simulink model "S_ELECTRO2025_V1"  (R2017a)
settings: Solver=VariableStepAuto  StartTime=0.0  StopTime=4  FixedStep=1e-6  MaxStep=1e-4  RelTol=1e-3
values from neighbouring files (symbols this model uses):
  Cdc = 470e-6    (= 0.00047)    [M_ELECTRO2025_V1.m]
  Cpv = 1e-6    (= 1e-06)    [M_ELECTRO2025_V1.m]
  Fred = fs    (= 60)    [M_ELECTRO2025_V1.m]
  fs = 60    [M_ELECTRO2025_V1.m]
  Icc_calc = In/(5/100)    [M_ELECTRO2025_V1.m]
  Irr_in = 0    [M_ELECTRO2025_V1.m]
  K1y2md = Kmd(1:end-1)    [M_ELECTRO2025_V1.m]
  KI2 = Ki2*Ts4    [M_ELECTRO2025_V1.m]
  KI4 = Ki4*Ts4    [M_ELECTRO2025_V1.m]
  KI5 = Ki5*Ts_inv    (= 0.17765287922)    [M_ELECTRO2025_V1.m]
  Kimd = -Kmd(end)    [M_ELECTRO2025_V1.m]
  KP2 = Kp2-KI2/2    [M_ELECTRO2025_V1.m]
  KP4 = Kp4-KI4/2    [M_ELECTRO2025_V1.m]
  KP5 = Kp5*Ts_inv-KI5/2    (= -0.0874937760062)    [M_ELECTRO2025_V1.m]
  L = 68.2729*Lmin    (= 0.100000049318)    [M_ELECTRO2025_V1.m]
  Linv = 0.0133    [M_ELECTRO2025_V1.m]
  Rinv = 0.0417    [M_ELECTRO2025_V1.m]
  S = 10e3*3/2    (= 15000)    [M_ELECTRO2025_V1.m]
  Ts1 = 1/Fs    (= 0.0002)    [M_ELECTRO2025_V1.m]
  Ts4 = 1/(4*Fc)    (= 0.000125)    [M_ELECTRO2025_V1.m]
  Ts_inv = 1/(100*Fc)    (= 5e-06)    [M_ELECTRO2025_V1.m]
  vdc = 1000    [M_ELECTRO2025_V1.m]
  vdc_ref = vdc    (= 1000)    [M_ELECTRO2025_V1.m]
  Vf = VL/sqrt(3)    [M_ELECTRO2025_V1.m]
  VL = (381.051/2)    (= 190.5255)    [M_ELECTRO2025_V1.m]
undefined symbols (not defined in the file or in its folder): DiscIntNeverNeededParam, sigbuilder_block
undefined symbols (not defined in the file): Fs, Ucmax
libraries: powerlib x22, powerlib_meascontrol x10, simulink x3, dsparch4 x3, re_lib x1
settings Model: Creator=dricl  LastModifiedBy=dricl

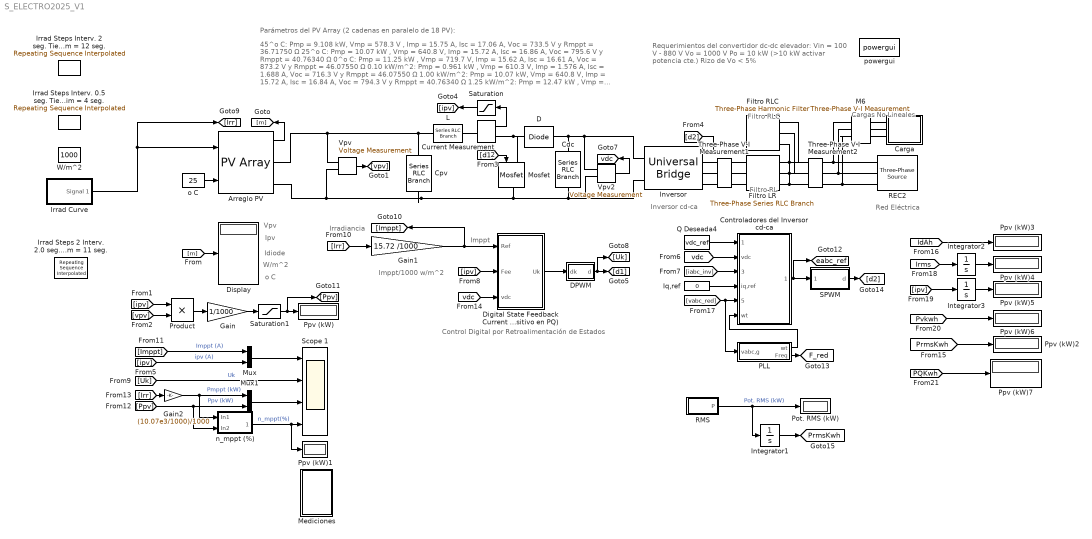
== system S_ELECTRO2025_V1 ==
  note: Control Digital por Retroalimentación de Estados
  note: Irradiancia
  note: Imppt/1000 w/m^2
  note: Imppt
  note: o C
  note: Idiode
  note: Ipv
  note: Vpv
  note: Requerimientos del convertidor dc-dc elevador:
      | Vin = 100 V - 880 V
      | Vo = 1000 V
      | Po = 10 kW (>10 kW activar potencia cte.)
      | Rizo de Vo < 5%
  note: Parámetros del PV Array (2 cadenas en paralelo de 18 PV):
  note: 45^o C: Pmp = 9.108 kW, Vmp = 578.3 V , Imp = 15.75 A, Isc = 17.06 A, Voc = 733.5 V y Rmppt = 36.71750 Ω
      | 25^o C: Pmp = 10.07 kW , Vmp = 640.8 V, Imp = 15.72 A, Isc = 16.86 A, Voc = 795.6 V y Rmppt = 40.76340 Ω
      | 0^o C: Pmp = 11.25 kW , Vmp = 719.7 V, Imp = 15.62 A, Isc = 16.61 A, Voc = 873.2 V y Rmppt = 46.07550 Ω
      | 0.10 kW/m^2: Pmp = 0.961 kW , Vmp = 610.3 V, Imp = 1.576 A, Isc = 1.688 A, Voc = 716.3 V y Rmppt = 46.07550 Ω
      | 1.00 kW/m^2: Pmp = 10.07 kW, Vmp = 640.8 V, Imp = 15.72 A, Isc = 16.84 A, Voc = 794.3 V y Rmppt = 40.76340 Ω
      | 1.25 kW/m^2: Pmp = 12.47 kW , Vmp = 636.0 V, Imp = 19.60 A, Isc = 19.60 A, Voc = 802.6 V y Rmppt = 32.44900 Ω
  note: W/m^2
  note: Red Eléctrica
  note: Filtro RL
  note: Inversor cd-ca
  note: Cargas No Lineales
  note: Filtro RLC
  Arreglo PV : re_lib/Solar/PV Array  Npar=No_Cadenas_Paralelo  Nser=No_Modulos_PorCadena  PlotType=array @ 1000 W/m2 & specified temperatures  S_vec=[ 1250 1000 100 ]  Temp_C_vec="[ 45 25  0]"  ModuleName=Canadian Solar CS6X-280P  PlotWhenSelected=off  Pm=279.816  Ncell=72  Voc=44.2  Isc=8.42  Vm=35.6  Im=7.86  beta_Voc_pc=-0.39  alpha_Isc_pc=0.06  beta_Voc=-0.17238  alpha_Isc=0.005052  IL=8.4417  I0=7.7188e-10  nI=1.0345  Rsh=300.2269  Rs=0.38773  BAL=off  Tc=1e-6  Tfilter=5e-5
  Carga : Subsystem
  Cdc : powerlib/Elements/Series RLC Branch  LConnTagsString=__new0  RConnTagsString=__new0  BranchType=C  Resistance=0.01  Inductance=1e-3  SetiL0=off  InitialCurrent=0  Capacitance=Cdc  Setx0=off  InitialVoltage=vdc_ref  Measurements=None
  Controladores del Inversor cd-ca : Subsystem
  Cpv : powerlib/Elements/Series RLC Branch  LConnTagsString=__new0  RConnTagsString=__new0  BranchType=C  Resistance=0.01  Inductance=1e-3  SetiL0=off  InitialCurrent=0  Capacitance=Cpv  Setx0=off  InitialVoltage=640.8  Measurements=None
  Current Measurement2 : powerlib/Measurements/Current Measurement  PhasorSimulation=off  OutputType=Complex  PSBequivalent=0
  D : powerlib/Power Electronics/Diode  Ron=0.001  Lon=0  Vf=0  IC=0  UseSnubber=0  Rs=500  Cs=250e-9  Measurements=off
  DPWM : Subsystem  AncestorBlock=plecslib_extras2/Modulators/Symmetrical PWM  mask(Symmetrical PWM){sampling=Natural (carrier starts with 0), fc=Fs, offset=0, input_limits=[0 Ucmax], output_values=[0 1]}
      mask prompts: fc "Carrier frequency (Hz):"; offset "Carrier offset (p.u.):"; input_limits "Input limits [min max]:"; output_values "Output values [off on]:"
      mask help: PWM generator with a symmetrical triangular carrier. If the input is a vector, the output is also a vector of the same width.
      mask init:
      | if numel(fc)>1 || fc<=0,
      |   error('Carrier frequency must be a positive scalar.');
      | end
      | if numel(offset)>1 || offset<0 || offset>=1,
      |   error('Carrier offset must be a scalar in the range [0; 1/fc[.');
      | end
      | if sampling == 1,
      |   offset = mod(offset+.75, 1);
      | end
      | 
      | si = [.5 mod(offset, .5)]/fc;
      mask Help: eval('plecs(''help'', ''symmetricalpwm.html'')')
      mask TypeOptions sampling: Natural (carrier starts with 0) | Natural (carrier starts with 1) | Regular (double edge) | Regular (single edge)
  "Digital State Feedback Current Controller n_mppt = 88.18%, ta(2%) = 0.4 s con Steps de Irrad Interv. 2 Seg. n_mppt = 97.01%, ta(2%) = 0.1 s con Steps de Irrad Interv. 2 Seg. n_mppt = 86.2%, ta(2%) = 0.4 s con Steps de Irrad Interv. 0.5 Seg. n_mppt = 93.3%, ta(2%) = 0.1 s con Steps de Irrad Interv. 0.5 Seg. n_mppt = 96.15%, ta(2%) = 0.1 s con Curva de Irrad ta(2%) de 0.1 s se obtiene el ta de F-Tsukmam n_mppt = 89.31%, ta(2%) = 0.0692 s con Steps de Irrad Interv. 0.5 Seg. Menor ta y tr: mayor n_mppt pero genera mayor MP en id (impacto negativo PQ). Si se mantiene ta y se incrementa tr la n_mppt se mantiene al mismo tiempo que se mitigan los MP en id (impacto positivo en PQ)  " : Subsystem
  Display : Display
  Filtro LR : powerlib/Elements/Three-Phase Series RLC Branch  LConnTagsString=A|B|C  RConnTagsString=A|B|C  BranchType=RL  Resistance=Rinv  Inductance=Linv  Capacitance=1e-6  Measurements=None
  Filtro RLC : powerlib/Elements/Three-Phase Harmonic Filter  LConnTagsString=A|B|C  FilterType=Single-tuned  FilterConnection=Y (grounded)  ParNom=[VL fs]  Qc=S*0.001  Fr=[31.42*60]  Frd=[40*fs 80*fs]  Q=5  Measurements=None
      settings: AttributesFormatString=\n  SourceProductName=Simscape Power Systems  SourceProductBaseCode=PS
  Gain : Gain  Gain=1/1000
  Gain1 : Gain  Gain=15.72 /1000
  Gain2 : Gain  Gain=(10.07e3/1000)/1000
  Integrator1 : Integrator  ZeroCross=off
  Integrator2 : Integrator  ZeroCross=off
  Integrator3 : Integrator  ZeroCross=off
  Inversor : powerlib/Power Electronics/Universal Bridge  Arms=3  SnubberResistance=1e5  SnubberCapacitance=inf  Device=IGBT / Diodes  Ron=1e-3  Lon=0  ForwardVoltages="[  0  0  ]"  ForwardVoltage=0  GTOparameters=[ 10e-6 , 20e-6 ]  IGBTparameters=[ 1e-6 , 2e-6 ]  Measurements=None  Measurements_2=None  converterType=Rectifier
  Iq,ref : Constant  Value=0  SampleTime=Ts4
  Irrad Curve : Subsystem  Tag=STV Subsys  LoadFcn=sigbuilder_block('load');  StartFcn=sigbuilder_block('start');  StopFcn=sigbuilder_block('stop');  ClipboardFcn=sigbuilder_block('clipboard');  mask(Sigbuilder block){tuvar=[0:10]}
      mask help: Simulink:masks:SigbuilderBlock_MD
      mask init:
      | if ~strcmp(get_param(bdroot(gcbh),'SimulationStatus'),'stopped') tuvar = sigbuilder_block('maskInit'); end
      settings: CopyFcn=sigbuilder_block('copy');  DeleteFcn=sigbuilder_block('delete');  ModelCloseFcn=sigbuilder_block('modelClose');  PreSaveFcn=sigbuilder_block('preSave');  PauseFcn=sigbuilder_block('pause');  ContinueFcn=sigbuilder_block('continue');  NameChangeFcn=sigbuilder_block('namechange');  OpenFcn=sigbuilder_block('open',[220.2 153.6 550.8 361.2 ]);  CloseFcn=sigbuilder_block('close');
      mask Display: plot(0, 0, 100, 100,[2, 2, 32, 32, 2], [68, 8, 8, 68, 68],[32, 2], [38, 38], [32, 19, 2],[53, 60, 44], [32, 17, 17, 2],[16, 16, 31, 31]);txt = getActiveGroup(gcbh);text(2, 100, txt,'verticalAlignment', 'top');
  Irrad Steps Interv. 0.5 seg. Tiempo sim = 4 seg. : simulink/Sources/Repeating Sequence Interpolated  OutValues=[Irr_in Irr_in 1000 1000 Irr_in Irr_in (Irr_in+1000)/2 (Irr_in+1000)/2 1000 1000 (Irr_in+1000)/2 (Irr_in+1000)/2 Irr_in Irr_in].'  TimeValues=[0 1/2 1.0001/2 2/2 2.0001/2 3/2 3.0001/2 4/2 4.001/2 5/2 5.0001/2 6/2 6.0001/2 7/2].'  LookUpMeth=Interpolation-Use End Values  tsamp=0.01  OutMin=[]  OutMax=[]  OutDataTypeStr=double  OutputDataTypeScalingMode=double  OutDataType=fixdt(0,8)  OutScaling=2^-10
  Irrad Steps Interv. 2 seg. Tiempo sim = 12 seg. : simulink/Sources/Repeating Sequence Interpolated  OutValues=[Irr_in Irr_in 1000 1000 Irr_in Irr_in (Irr_in+1000)/2 (Irr_in+1000)/2 1000 1000 (Irr_in+1000)/2 (Irr_in+1000)/2 Irr_in Irr_in].'  TimeValues=[0 1 1.001 3 3.001 5 5.001 7 7.001 9 9.001 11 11.001 12].'  LookUpMeth=Interpolation-Use End Values  tsamp=0.01  OutMin=[]  OutMax=[]  OutDataTypeStr=double  OutputDataTypeScalingMode=double  OutDataType=fixdt(0,8)  OutScaling=2^-10
  Irrad Steps 2 Interv. 2.0 seg. Tiempo sim = 11 seg. : simulink/Sources/Repeating Sequence Interpolated  OutValues=[0 0 1000 1000 500 500 300 300 600 600 1000 1000].'  TimeValues=[0 1.0 1.01 3 3.001 5 5.001 7.0 7.001 9 9.001 11.0].'  LookUpMeth=Interpolation-Use End Values  tsamp=0.01  OutMin=[]  OutMax=[]  OutDataTypeStr=double  OutputDataTypeScalingMode=double  OutDataType=fixdt(0,8)  OutScaling=2^-10
  L : powerlib/Elements/Series RLC Branch  LConnTagsString=__new0  RConnTagsString=__new0  BranchType=L  Resistance=40.76340  Inductance=L  SetiL0=off  InitialCurrent=0  Capacitance=1e-6  Setx0=off  InitialVoltage=0  Measurements=None
  M6 : powerlib/Measurements/Three-Phase V-I Measurement  VoltageMeasurement=phase-to-ground  SetLabelV=on  LabelV=vabc_nl_load  Vpu=off  VpuLL=off  CurrentMeasurement=yes  SetLabelI=on  LabelI=iabc_nl_load  Ipu=off  Pbase=3.6e6  Vbase=0.69e3  OutputType=Magnitude  PhasorSimulation=off  PSBequivalent=0
  Mediciones : Subsystem
  Mosfet : powerlib/Power Electronics/Mosfet  Ron=0.001  Lon=0  Rd=0  Vfd=0  IC=0  Rs=1e5  Cs=inf  Measurements=off
  Mux : Mux  Inputs=2
  Mux1 : Mux  Inputs=2
  PLL : Subsystem
  Pot. RMS (kW) : Display
  Ppv (kW){,1..7} (8 alike) : Display
  Product : Product
  Q Deseada4 : Constant  Value=vdc_ref  SampleTime=Ts4
  REC2 : powerlib/Electrical Sources/Three-Phase Source  InternalConnection=Yg  VoltagePhases=on  Voltage=VL  PhaseAngle=0  Voltage_phases=[VL/sqrt(3) VL/sqrt(3) VL/sqrt(3)]  PhaseAngles_phases=[0 -120 +120]  Frequency=Fred  NonIdealSource=on  SpecifyImpedance=on  Resistance=25e3^2/10e6/5  Inductance=25e3^2/10e6/377  ShortCircuitLevel=Icc_calc*2  BaseVoltage=VL  XRratio=7  BusType=swing  Pref=-500e3  Qref=0  Prefabc=[10e3, 10e3, 10e3]  Qrefabc=[0, 0, 0]  Qmin=-inf  Qmax=inf
  RMS : Subsystem
  SPWM : Subsystem
  Saturation : Saturate  UpperLimit=inf  LowerLimit=0
  Saturation1 : Saturate  UpperLimit=inf  LowerLimit=0
  Scope 1 : Scope  NumInputPorts=4
  Three-Phase V-I Measurement1 : powerlib/Measurements/Three-Phase V-I Measurement  VoltageMeasurement=phase-to-ground  SetLabelV=on  LabelV=vabc_inv  Vpu=off  VpuLL=off  CurrentMeasurement=yes  SetLabelI=on  LabelI=iabc_inv  Ipu=off  Pbase=100e6  Vbase=500e3  OutputType=Complex  PhasorSimulation=off  PSBequivalent=0
  Three-Phase V-I Measurement2 : powerlib/Measurements/Three-Phase V-I Measurement  VoltageMeasurement=phase-to-ground  SetLabelV=on  LabelV=vabc_red  Vpu=off  VpuLL=off  CurrentMeasurement=yes  SetLabelI=on  LabelI=iabc_red  Ipu=off  Pbase=100e6  Vbase=500e3  OutputType=Complex  PhasorSimulation=off  PSBequivalent=0
  Vpv : powerlib/Measurements/Voltage Measurement  PhasorSimulation=off  OutputType=Complex  PSBequivalent=0
  Vpv2 : powerlib/Measurements/Voltage Measurement  PhasorSimulation=off  OutputType=Complex  PSBequivalent=0
  W/m^2 : Constant  Value=1000
  n_mppt (%) : Subsystem
  o C : Constant  Value=25
  powergui : powerlib/powergui  Priority=1  SimulationMode=Continuous  SampleTime=1e-6  frequency=60  Iterations=50  frequencyindice=0  Pbase=100e6  ErrMax=1e-4  UnitsV=kV  UnitsW=MW  buscounter=0  FunctionMessages=off  echomessages=off  EnableUseOfTLC=off  CurrentSourceSwitches=off  DisableSnubberDevices=off  DisableRonSwitches=off  DisableVfSwitches=off  DisplayEquations=off  SolverType=Tustin/Backward Euler (TBE)  Interpol=off  ExternalGateDelay=off  methode=off  Ts=100  x0status=blocks  SPID=on  SwTol=0  HookPort=off  RestoreLinks=warning  ResistiveCurrentMeasurement=off  Frange=[0:2:500]  Ylog=off  Xlog=on  ShowGrid=off  save=off  variable=ZData  structure=0  ZoomFFT=off  StartTime=0.0  cycles=1  DisplayStyle=1  fundamental=60  FreqAxis=off  MaxFrequency=1000  frequencyindicesteady=1  RmsSteady=1  display=off
  tag scope: F_red=global, PrmsKwh=global, eabc_ref=global, vdc=global
  wires:
  o C/1 -> Arreglo PV/2
  Arreglo PV/1 -> [m]
  [m] -> Display/1
  Vpv/1 -> [vpv]
  [ipv] -> Product/1
  [vpv] -> Product/2
  Product/1 -> Gain/1
  Gain/1 -> Saturation1/1
  Current Measurement2/1 -> Saturation/1
  Vpv2/1 -> [vdc]
  [d1] -> Mosfet/1
  [Irr] -> Gain1/1
  [ipv] -> Mux/2  "ipv (A)"
  [Imppt] -> Mux/1  "Imppt (A)"
  [Ppv] -> n_mppt (%)/2(In2), Mux1/2  "Ppv (kW)"
  [Irr] -> Gain2/1
  Gain2/1 -> n_mppt (%)/1(In1), Mux1/1  "Pmppt (kW)"
  Gain1/1 -> "Digital State Feedback Current Controller n_mppt = 88.18%, ta(2%) = 0.4 s con Steps de Irrad Interv. 2 Seg. n_mppt = 97.01%, ta(2%) = 0.1 s con Steps de Irrad Interv. 2 Seg. n_mppt = 86.2%, ta(2%) = 0.4 s con Steps de Irrad Interv. 0.5 Seg. n_mppt = 93.3%, ta(2%) = 0.1 s con Steps de Irrad Interv. 0.5 Seg. n_mppt = 96.15%, ta(2%) = 0.1 s con Curva de Irrad ta(2%) de 0.1 s se obtiene el ta de F-Tsukmam n_mppt = 89.31%, ta(2%) = 0.0692 s con Steps de Irrad Interv. 0.5 Seg. Menor ta y tr: mayor n_mppt pero genera mayor MP en id (impacto negativo PQ). Si se mantiene ta y se incrementa tr la n_mppt se mantiene al mismo tiempo que se mitigan los MP en id (impacto positivo en PQ)  "/1(Ref), [Imppt]
  [ipv] -> "Digital State Feedback Current Controller n_mppt = 88.18%, ta(2%) = 0.4 s con Steps de Irrad Interv. 2 Seg. n_mppt = 97.01%, ta(2%) = 0.1 s con Steps de Irrad Interv. 2 Seg. n_mppt = 86.2%, ta(2%) = 0.4 s con Steps de Irrad Interv. 0.5 Seg. n_mppt = 93.3%, ta(2%) = 0.1 s con Steps de Irrad Interv. 0.5 Seg. n_mppt = 96.15%, ta(2%) = 0.1 s con Curva de Irrad ta(2%) de 0.1 s se obtiene el ta de F-Tsukmam n_mppt = 89.31%, ta(2%) = 0.0692 s con Steps de Irrad Interv. 0.5 Seg. Menor ta y tr: mayor n_mppt pero genera mayor MP en id (impacto negativo PQ). Si se mantiene ta y se incrementa tr la n_mppt se mantiene al mismo tiempo que se mitigan los MP en id (impacto positivo en PQ)  "/2(Fee)
  [Uk] -> Scope 1/2  "Uk"
  n_mppt (%)/1(Out1) -> Ppv (kW)1/1, Scope 1/4  "n_mppt(%)"
  [d2] -> Inversor/1
  RMS/1(P) -> Integrator1/1, Pot. RMS (kW)/1  "Pot. RMS (kW)"
  [vabc_red] -> Controladores del Inversor cd-ca/5(vabc,red), PLL/1(vabc,g)
  PLL/1(wt) -> Controladores del Inversor cd-ca/6(wt)
  [iabc_inv] -> Controladores del Inversor cd-ca/3(iabc,inv)
  Controladores del Inversor cd-ca/1(eabc,ref) -> [eabc_ref], SPWM/1(eabc,ref)
  PLL/2(Freq) -> [F_red]
  Iq,ref/1 -> Controladores del Inversor cd-ca/4(iq,ref)
  [vdc] -> Controladores del Inversor cd-ca/2(vdc)
  SPWM/1(d) -> [d2]
  [vdc] -> "Digital State Feedback Current Controller n_mppt = 88.18%, ta(2%) = 0.4 s con Steps de Irrad Interv. 2 Seg. n_mppt = 97.01%, ta(2%) = 0.1 s con Steps de Irrad Interv. 2 Seg. n_mppt = 86.2%, ta(2%) = 0.4 s con Steps de Irrad Interv. 0.5 Seg. n_mppt = 93.3%, ta(2%) = 0.1 s con Steps de Irrad Interv. 0.5 Seg. n_mppt = 96.15%, ta(2%) = 0.1 s con Curva de Irrad ta(2%) de 0.1 s se obtiene el ta de F-Tsukmam n_mppt = 89.31%, ta(2%) = 0.0692 s con Steps de Irrad Interv. 0.5 Seg. Menor ta y tr: mayor n_mppt pero genera mayor MP en id (impacto negativo PQ). Si se mantiene ta y se incrementa tr la n_mppt se mantiene al mismo tiempo que se mitigan los MP en id (impacto positivo en PQ)  "/3(vdc)
  DPWM/1(d) -> [Uk], [d1]
  Mux1/1 -> Scope 1/3
  Mux/1 -> Scope 1/1
  Saturation/1 -> [ipv]
  Saturation1/1 -> [Ppv], Ppv (kW)/1
  Q Deseada4/1 -> Controladores del Inversor cd-ca/1(vdc,ref)
  [IdAh] -> Ppv (kW)3/1
  [Irms] -> Integrator2/1
  Integrator2/1 -> Ppv (kW)4/1
  [ipv] -> Integrator3/1
  Integrator3/1 -> Ppv (kW)5/1
  [Pvkwh] -> Ppv (kW)6/1
  Integrator1/1 -> [PrmsKwh]
  [PrmsKwh] -> Ppv (kW)2/1
  [PQKwh] -> Ppv (kW)7/1
  "Digital State Feedback Current Controller n_mppt = 88.18%, ta(2%) = 0.4 s con Steps de Irrad Interv. 2 Seg. n_mppt = 97.01%, ta(2%) = 0.1 s con Steps de Irrad Interv. 2 Seg. n_mppt = 86.2%, ta(2%) = 0.4 s con Steps de Irrad Interv. 0.5 Seg. n_mppt = 93.3%, ta(2%) = 0.1 s con Steps de Irrad Interv. 0.5 Seg. n_mppt = 96.15%, ta(2%) = 0.1 s con Curva de Irrad ta(2%) de 0.1 s se obtiene el ta de F-Tsukmam n_mppt = 89.31%, ta(2%) = 0.0692 s con Steps de Irrad Interv. 0.5 Seg. Menor ta y tr: mayor n_mppt pero genera mayor MP en id (impacto negativo PQ). Si se mantiene ta y se incrementa tr la n_mppt se mantiene al mismo tiempo que se mitigan los MP en id (impacto positivo en PQ)  "/1(Uk) -> DPWM/1(dk)
  Irrad Curve/1(Signal 1) -> [Irr], Arreglo PV/1
  connections:
  Current Measurement2/LConn1 -- L/RConn1
  Mosfet/LConn1 -- D/LConn1 -- Current Measurement2/RConn1
  Vpv2/LConn1 -- Inversor/RConn1 -- Cdc/LConn1 -- D/RConn1
  Vpv/LConn2 -- Inversor/RConn2 -- Vpv2/LConn2 -- Cdc/RConn1 -- Mosfet/RConn1 -- Cpv/RConn1 -- Arreglo PV/RConn2
  M6/LConn1 -- Three-Phase V-I Measurement2/RConn1 -- REC2/RConn1
  M6/LConn2 -- Three-Phase V-I Measurement2/RConn2 -- REC2/RConn2
  M6/LConn3 -- Three-Phase V-I Measurement2/RConn3 -- REC2/RConn3
  Filtro LR/RConn2 -- Three-Phase V-I Measurement2/LConn2 -- Filtro RLC/LConn2
  Filtro LR/RConn3 -- Three-Phase V-I Measurement2/LConn3 -- Filtro RLC/LConn3
  Filtro LR/RConn1 -- Three-Phase V-I Measurement2/LConn1 -- Filtro RLC/LConn1
  Three-Phase V-I Measurement1/RConn1 -- Filtro LR/LConn1
  Three-Phase V-I Measurement1/LConn1 -- Inversor/LConn1
  Three-Phase V-I Measurement1/RConn3 -- Filtro LR/LConn3
  Three-Phase V-I Measurement1/LConn3 -- Inversor/LConn3
  Three-Phase V-I Measurement1/RConn2 -- Filtro LR/LConn2
  Three-Phase V-I Measurement1/LConn2 -- Inversor/LConn2
  M6/RConn3 -- Carga/LConn3
  M6/RConn1 -- Carga/LConn1
  M6/RConn2 -- Carga/LConn2
  Cpv/LConn1 -- L/LConn1 -- Vpv/LConn1 -- Arreglo PV/RConn1

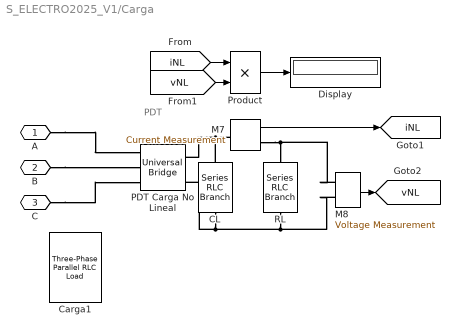
== system S_ELECTRO2025_V1/Carga ==
  note: PDT
  CL : powerlib/Elements/Series RLC Branch  LConnTagsString=__new0  RConnTagsString=__new0  BranchType=RC  Resistance=0.01  Inductance=1e-3  SetiL0=off  InitialCurrent=0  Capacitance=470e-6  Setx0=on  InitialVoltage=500  Measurements=None
  Carga1 : powerlib/Elements/Three-Phase Parallel RLC Load  LConnTagsString=A|B|C  Configuration=Y (grounded)  NominalVoltage=120  Vabc=[VL/sqrt(3) VL/sqrt(3) VL/sqrt(3)]  Vabcp=[1e3 1e3 1e3]  NominalFrequency=fs  UnbalancedPower=on  ActivePower=S/1  InductivePower=0  CapacitivePower=0  Pabc=[(S*2/3)/3 (S*2/3)/3 (S*2/3)/3]*0.5  QLabc=[(S*2/3)/3 (S*2/3)/3 (S*2/3)/3]*0.5  QCabc=[(S*2/3)/3 (S*2/3)/3 (S*2/3)/3]*0.0  Pabcp=[10e3 9e3 11e3]  QLabcp=[100 90 110]  QCabcp=[100 90 110]  Measurements=None  LoadType=constant Z
  Display : Display
  M7 : powerlib/Measurements/Current Measurement  PhasorSimulation=off  OutputType=Complex  PSBequivalent=0
  M8 : powerlib/Measurements/Voltage Measurement  PhasorSimulation=off  OutputType=Complex  PSBequivalent=0
  PDT Carga No Lineal : powerlib/Power Electronics/Universal Bridge  Arms=3  SnubberResistance=1e5  SnubberCapacitance=inf  Device=Diodes  Ron=0.07  Lon=0  ForwardVoltages="[  0  0  ]"  ForwardVoltage=0.7  GTOparameters=[ 10e-6 , 20e-6 ]  IGBTparameters=[ 1e-6 , 2e-6 ]  Measurements=None  Measurements_2=None  converterType=Rectifier
  Product : Product
  RL : powerlib/Elements/Series RLC Branch  LConnTagsString=__new0  RConnTagsString=__new0  BranchType=RL  Resistance=5  Inductance=1  SetiL0=on  InitialCurrent=0  Capacitance=2200e-6  Setx0=on  InitialVoltage=0  Measurements=None
  A : PMIOPort  Port=1  Side=Left
  B : PMIOPort  Port=2  Side=Left
  C : PMIOPort  Port=3  Side=Left
  tag scope: iNL=global, vNL=global
  wires:
  M7/1 -> [iNL]
  M8/1 -> [vNL]
  [iNL] -> Product/1
  [vNL] -> Product/2
  Product/1 -> Display/1
  connections:
  RL/RConn1 -- M8/LConn2 -- CL/RConn1 -- PDT Carga No Lineal/RConn2
  M8/LConn1 -- RL/LConn1 -- M7/RConn1
  M7/LConn1 -- CL/LConn1 -- PDT Carga No Lineal/RConn1
  A/RConn1 -- PDT Carga No Lineal/LConn1
  B/RConn1 -- PDT Carga No Lineal/LConn2
  C/RConn1 -- PDT Carga No Lineal/LConn3

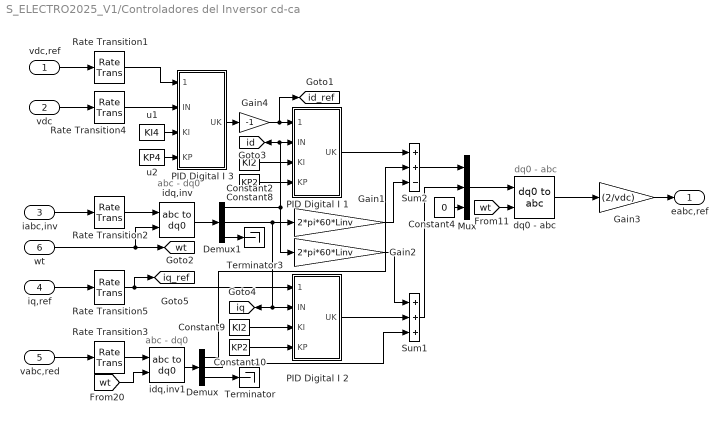
== system S_ELECTRO2025_V1/Controladores del Inversor cd-ca ==
  note: dq0 - abc
  note: abc - dq0
  note: abc - dq0
  vdc,ref : Inport
  vdc : Inport  Port=2
  iabc,inv : Inport  Port=3
  iq,ref : Inport  Port=4
  vabc,red : Inport  Port=5
  wt : Inport  Port=6
  Constant10 : Constant  Value=KP2  SampleTime=Ts4
  Constant2 : Constant  Value=KI2  SampleTime=Ts4
  Constant4 : Constant  Value=0  SampleTime=Ts4
  Constant8 : Constant  Value=KP2  SampleTime=Ts4
  Constant9 : Constant  Value=KI2  SampleTime=Ts4
  Demux : Demux  Outputs=3
  Demux1 : Demux  Outputs=3
  Gain1 : Gain  Gain=2*pi*60*Linv
  Gain2 : Gain  Gain=2*pi*60*Linv
  Gain3 : Gain  Gain=(2/vdc)
  Gain4 : Gain  Gain=-1
  Mux : Mux  Inputs=3
  PID Digital I 1 : MATLAB Function  TreatAsAtomicUnit=on
  PID Digital I 2 : MATLAB Function  TreatAsAtomicUnit=on
  PID Digital I 3 : MATLAB Function  TreatAsAtomicUnit=on
  Rate Transition{1..5} (5 alike) : RateTransition  OutPortSampleTime=Ts4
  Sum1 : Sum  Inputs=+++
  Sum2 : Sum  Inputs=++-
  Terminator : Terminator
  Terminator3 : Terminator
  dq0 - abc : powerlib_meascontrol/Transformations/dq0 to abc  Alignment=90 degrees behind phase A axis
  idq,inv : powerlib_meascontrol/Transformations/abc to dq0  Alignment=90 degrees behind phase A axis
  idq,inv1 : powerlib_meascontrol/Transformations/abc to dq0  Alignment=90 degrees behind phase A axis
  u1 : Constant  Value=KI4  SampleTime=Ts4
  u2 : Constant  Value=KP4  SampleTime=Ts4
  eabc,ref : Outport
  tag scope: id=global, id_ref=global, iq=global, iq_ref=global, wt=global
  wires:
  vabc,red/1 -> Rate Transition3/1
  Rate Transition4/1 -> PID Digital I 3/2(IN)
  Demux/2 -> Sum1/3
  Demux1/2 -> PID Digital I 2/2(IN), [iq], Gain1/1
  PID Digital I 1/1(UK) -> Sum2/1
  Gain4/1 -> [id_ref], PID Digital I 1/1(IN_ref)
  Sum1/1 -> Mux/2
  Mux/1 -> dq0 - abc/1
  Constant4/1 -> Mux/3
  [wt] -> dq0 - abc/2
  Demux/3 -> Terminator/1
  Demux1/1 -> [id], PID Digital I 1/2(IN), Gain2/1
  Constant8/1 -> PID Digital I 1/4(KP)
  Rate Transition5/1 -> [iq_ref], PID Digital I 2/1(IN_ref)
  idq,inv1/1 -> Demux/1
  iq,ref/1 -> Rate Transition5/1
  idq,inv/1 -> Demux1/1
  Constant9/1 -> PID Digital I 2/3(KI)
  u1/1 -> PID Digital I 3/3(KI)
  vdc,ref/1 -> Rate Transition1/1
  Constant10/1 -> PID Digital I 2/4(KP)
  vdc/1 -> Rate Transition4/1
  Constant2/1 -> PID Digital I 1/3(KI)
  iabc,inv/1 -> Rate Transition2/1
  Rate Transition2/1 -> idq,inv/1
  Demux1/3 -> Terminator3/1
  Rate Transition3/1 -> idq,inv1/1
  u2/1 -> PID Digital I 3/4(KP)
  PID Digital I 2/1(UK) -> Sum1/2
  Sum2/1 -> Mux/1
  Demux/1 -> Sum2/2
  Gain2/1 -> Sum1/1
  Gain1/1 -> Sum2/3
  [wt] -> idq,inv1/2
  wt/1 -> [wt], idq,inv/2
  dq0 - abc/1 -> Gain3/1
  PID Digital I 3/1(UK) -> Gain4/1
  Rate Transition1/1 -> PID Digital I 3/1(IN_ref)
  Gain3/1 -> eabc,ref/1

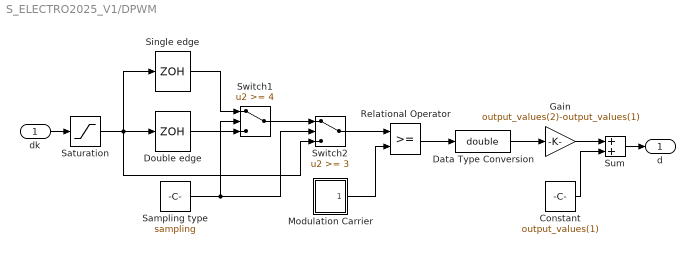
== system S_ELECTRO2025_V1/DPWM ==
  dk : Inport
  Constant : Constant  Value=output_values(1)
  Data Type Conversion : DataTypeConversion  OutDataTypeStr=double  SaturateOnIntegerOverflow=on  RndMeth=Zero
  Double edge : ZeroOrderHold  SampleTime=si
  Gain : Gain  Gain=output_values(2)-output_values(1)  SaturateOnIntegerOverflow=on  OutDataTypeStr=Inherit: Same as input  ParamDataTypeStr=Inherit: Same as input
  Modulation Carrier : Subsystem  mask(Symmetric Triangle Generator){fc=fc, offset=mod(offset+.5, 1), range=input_limits}
      mask prompts: fc "Carrier frequency (Hz):"; offset "Carrier offset (p.u.):"; range "Signal range [min max]:"
      mask help: Generates a symmetrical triangular signal with output values between 0 and 1. The block forces the Simulink solver to output all tips of the signal. The output can therefore be used as a carrier signal for PWM.
      mask init:
      | if numel(fc)>1 || fc<=0,
      |   error('Carrier frequency must be a positive scalar.');
      | end
      | if numel(offset)>1 || offset<0 || offset>=1,
      |   error('Carrier offset must be a scalar in the interval [0; 1[.');
      | end
      | if numel(range)~=2,
      |   error('Signal range must be a two-element vector.')
      | end
      | if range(1)>=range(2),
      |   error('Signal range must be specified as [min max].')
      | end
      | 
      | carrier_t = [0 offset mod(1/2+offset, 1) 1]/fc;
      | carrier_v0 = 1-2*abs(offset-.5);
      | carrier_v = range(1)+[carrier_v0 0 1 carrier_v0]*diff(range);
      | [carrier_t, idx] = unique(carrier_t);
      | carrier_v = carrier_v(idx);
      | si = [.5 mod(offset, .5)]/fc;
      | 
      | L = length(carrier_t);
      | disp_seq_t = repmat(carrier_t(:),1,3) + ones(L,1)*[0,1,2]/fc;
      | disp_seq_v = repmat(carrier_v(:),1,3);
      mask Display: plot(disp_seq_t, disp_seq_v)
  Relational Operator : RelationalOperator  RndMeth=Nearest  InputSameDT=on
  Sampling type : Constant  Value=sampling
  Saturation : Saturate  UpperLimit=input_limits(2)  LowerLimit=input_limits(1)
  Single edge : ZeroOrderHold  SampleTime=[1 offset]/fc
  Sum : Sum  SaturateOnIntegerOverflow=on  InputSameDT=on  OutDataTypeStr=Inherit: Same as first input
  Switch1 : Switch  Threshold=4  SaturateOnIntegerOverflow=on  InputSameDT=on
  Switch2 : Switch  Threshold=3  SaturateOnIntegerOverflow=on  InputSameDT=on
  d : Outport
  wires:
  Data Type Conversion/1 -> Gain/1
  Constant/1 -> Sum/2
  Gain/1 -> Sum/1
  Sum/1 -> d/1
  Relational Operator/1 -> Data Type Conversion/1
  Switch2/1 -> Relational Operator/1
  Sampling type/1 -> Switch1/2, Switch2/2
  Single edge/1 -> Switch1/1
  Saturation/1 -> Double edge/1, Single edge/1, Switch2/3
  dk/1 -> Saturation/1
  Modulation Carrier/1(Out) -> Relational Operator/2
  Switch1/1 -> Switch2/1
  Double edge/1 -> Switch1/3

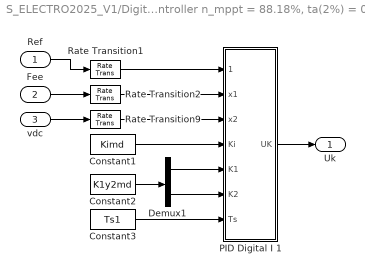
== system S_ELECTRO2025_V1/Digital State Feedback Current Controller n_mppt = 88.18%, ta(2%) = 0.4 s con Steps de Irrad Interv. 2 Seg. n_mppt = 97.01%, ta(2%) = 0.1 s con Steps de Irrad Interv. 2 Seg. n_mppt = 86.2%, ta(2%) = 0.4 s con Steps de Irrad Interv. 0.5 Seg. n_mppt = 93.3%, ta(2%) = 0.1 s con Steps de Irrad Interv. 0.5 Seg. n_mppt = 96.15%, ta(2%) = 0.1 s con Curva de Irrad ta(2%) de 0.1 s se obtiene el ta de F-Tsukmam n_mppt = 89.31%, ta(2%) = 0.0692 s con Steps de Irrad Interv. 0.5 Seg. Menor ta y tr: mayor n_mppt pero genera mayor MP en id (impacto negativo PQ). Si se mantiene ta y se incrementa tr la n_mppt se mantiene al mismo tiempo que se mitigan los MP en id (impacto positivo en PQ)   ==
  Ref : Inport
  Fee : Inport  Port=2
  vdc : Inport  Port=3
  Constant1 : Constant  Value=Kimd  SampleTime=Ts1
  Constant2 : Constant  Value=K1y2md  SampleTime=Ts1
  Constant3 : Constant  Value=Ts1  SampleTime=Ts1
  Demux1 : Demux  Outputs=2
  PID Digital I 1 : MATLAB Function  TreatAsAtomicUnit=on
  Rate Transition1 : RateTransition  OutPortSampleTime=Ts1
  Rate Transition2 : RateTransition  OutPortSampleTime=Ts1
  Rate Transition9 : RateTransition  OutPortSampleTime=Ts1
  Uk : Outport
  wires:
  Rate Transition9/1 -> PID Digital I 1/3(x2)
  Fee/1 -> Rate Transition2/1
  Ref/1 -> Rate Transition1/1
  vdc/1 -> Rate Transition9/1
  Rate Transition1/1 -> PID Digital I 1/1(x1_Ref)
  Rate Transition2/1 -> PID Digital I 1/2(x1)
  Constant3/1 -> PID Digital I 1/7(Ts)
  PID Digital I 1/1(UK) -> Uk/1
  Constant2/1 -> Demux1/1
  Constant1/1 -> PID Digital I 1/4(Ki)
  Demux1/1 -> PID Digital I 1/5(K1)
  Demux1/2 -> PID Digital I 1/6(K2)

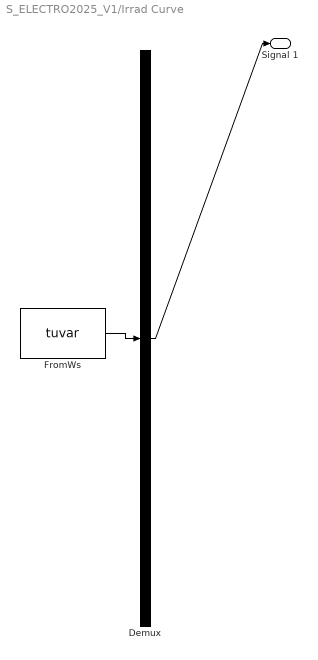
== system S_ELECTRO2025_V1/Irrad Curve ==
  Demux : Demux  Tag=STV Demux  Outputs=1
  FromWs : FromWorkspace  Tag=STV FromWs  VariableName=tuvar  SampleTime=0
      SigBuilderData=|
      | common.afterFinalStr = 'Extrapolate'
      | common.sampleTime = 0
      | dataSet.timeRange = [0 4]
      | dataSet.name = 'Group 1'
      | sbobj.Groups.Name = 'Group 1'
      | sbobj.Groups.Signals.Name = 'Signal 1'
      | sbobj.Groups.Signals.XData = [0 0.00416233090531 0.00832466181061 0.0124869927159 0.0166493236212 0.0208116545265 0.0249739854318 0.0291363163371 0.0332986472425 0.0374609781478 0.0416233090531 0.0457856399584 ... (962 elements, 1x962)]
      | sbobj.Groups.Signals.YData = [2.47122187864 2.47122187864 2.47122187864 2.47122187864 2.47122187864 2.47122187864 2.47122187864 2.47122187864 2.47122187864 2.47121149505 2.47121149505 2.47121149505 ... (962 elements, 1x962)]
      | sbobj.Groups.TimeRange = [0 4]
  Signal 1 : Outport  Tag=STV Outport
  wires:
  FromWs/1 -> Demux/1
  Demux/1 -> Signal 1/1

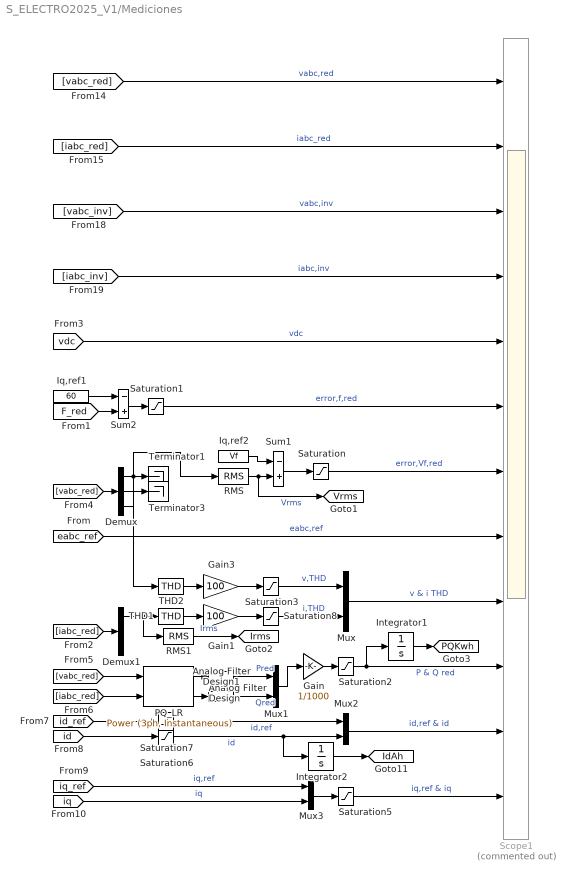
== system S_ELECTRO2025_V1/Mediciones ==
  Analog Filter Design : dsparch4/Analog Filter Design  method=Butterworth  filttype=Lowpass  N=8  Wlo=4000  Whi=80  Rp=2  Rs=40
  Analog Filter Design1 : dsparch4/Analog Filter Design  method=Butterworth  filttype=Lowpass  N=8  Wlo=4000  Whi=80  Rp=2  Rs=40
  Demux : Demux  Outputs=3
  Demux1 : Demux  Outputs=3
  Gain : Gain  Gain=1/1000
  Gain1 : Gain  Gain=100
  Gain3 : Gain  Gain=100
  Integrator1 : Integrator  ZeroCross=off
  Integrator2 : Integrator  ZeroCross=off
  Iq,ref1 : Constant  Value=60  SampleTime=Ts4
  Iq,ref2 : Constant  Value=Vf  SampleTime=Ts4
  Mux{,1..3} (4 alike) : Mux  Inputs=2
  PQ_LR : powerlib_meascontrol/Measurements/Power (3ph, Instantaneous)
      settings: SourceProductName=Simscape Power Systems
  RMS : powerlib_meascontrol/Measurements/RMS  TrueRMS=on  Freq=60  RMSInit=0  Ts=0
  RMS1 : powerlib_meascontrol/Measurements/RMS  TrueRMS=on  Freq=60  RMSInit=0  Ts=0
  Saturation : Saturate  UpperLimit=5.5  LowerLimit=-5.5
  Saturation1 : Saturate  UpperLimit=1  LowerLimit=-1
  Saturation2 : Saturate  UpperLimit=20  LowerLimit=0
  Saturation3 : Saturate  UpperLimit=20  LowerLimit=0
  Saturation5 : Saturate  UpperLimit=100  LowerLimit=0
  Saturation6 : Saturate  UpperLimit=inf  LowerLimit=0
  Saturation7 : Saturate  UpperLimit=inf  LowerLimit=0
  Saturation8 : Saturate  UpperLimit=20  LowerLimit=0
  Scope1 : Scope  Commented=on  NumInputPorts=12
  Sum1 : Sum  Inputs=-+
  Sum2 : Sum  Inputs=-+
  THD1 : powerlib_meascontrol/Measurements/THD  Freq=60  Ts=0
  THD2 : powerlib_meascontrol/Measurements/THD  Freq=60  Ts=0
  Terminator1 : Terminator
  Terminator3 : Terminator
  tag scope: IdAh=global, Irms=global, PQKwh=global, Vrms=global
  wires:
  Saturation/1 -> Scope1/7  "error,Vf,red"
  [vabc_red] -> Scope1/1  "vabc,red"
  [eabc_ref] -> Scope1/8  "eabc,ref"
  [iabc_red] -> Scope1/2  "iabc_red"
  Demux/1 -> THD2/1, RMS/1
  [vdc] -> Scope1/5  "vdc"
  [iabc_inv] -> Scope1/4  "iabc,inv"
  [vabc_inv] -> Scope1/3  "vabc,inv"
  Sum1/1 -> Saturation/1
  RMS/1 -> [Vrms], Sum1/2  "Vrms"
  Demux/2 -> Terminator3/1
  Demux/3 -> Terminator1/1
  [vabc_red] -> Demux/1
  [F_red] -> Sum2/2
  Iq,ref2/1 -> Sum1/1
  Iq,ref1/1 -> Sum2/1
  Saturation1/1 -> Scope1/6  "error,f,red"
  Sum2/1 -> Saturation1/1
  [iabc_red] -> Demux1/1
  Demux1/1 -> RMS1/1, THD1/1
  THD2/1 -> Gain3/1
  THD1/1 -> Gain1/1
  Mux/1 -> Scope1/9  "v & i THD"
  [vabc_red] -> PQ_LR/1
  [iabc_red] -> PQ_LR/2
  PQ_LR/1 -> Analog Filter Design/1
  Analog Filter Design/1 -> Mux1/1  "Pred"
  PQ_LR/2 -> Analog Filter Design1/1
  Analog Filter Design1/1 -> Mux1/2  "Qred"
  Saturation2/1 -> Integrator1/1, Scope1/10  "P & Q red"
  Gain/1 -> Saturation2/1
  Mux1/1 -> Gain/1
  Mux3/1 -> Saturation5/1
  [iq] -> Mux3/2  "iq"
  [id] -> Saturation6/1
  [iq_ref] -> Mux3/1  "iq,ref"
  [id_ref] -> Saturation7/1
  Mux2/1 -> Scope1/11  "id,ref & id"
  Saturation5/1 -> Scope1/12  "iq,ref & iq"
  RMS1/1 -> [Irms]  "Irms"
  Saturation6/1 -> Integrator2/1, Mux2/2  "id"
  Saturation7/1 -> Mux2/1  "id,ref"
  Gain3/1 -> Saturation3/1
  Saturation3/1 -> Mux/1  "v,THD"
  Saturation8/1 -> Mux/2  "i,THD"
  Gain1/1 -> Saturation8/1
  Integrator2/1 -> [IdAh]
  Integrator1/1 -> [PQKwh]

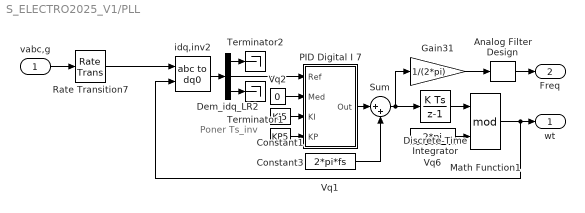
== system S_ELECTRO2025_V1/PLL ==
  note: Poner Ts_inv
  vabc,g : Inport
  Analog Filter Design : dsparch4/Analog Filter Design  method=Butterworth  filttype=Lowpass  N=8  Wlo=4000  Whi=80  Rp=2  Rs=40
  Constant1 : Constant  Value=KI5  SampleTime=Ts_inv
  Constant3 : Constant  Value=KP5  SampleTime=Ts_inv
  Dem_idq_LR2 : Demux  Outputs=3
  Discrete-Time Integrator : DiscreteIntegrator  InitialConditionSetting=State (most efficient)  SampleTime=Ts_inv  ICPrevOutput=DiscIntNeverNeededParam  ICPrevScaledInput=DiscIntNeverNeededParam
  Gain31 : Gain  Gain=1/(2*pi)  OutMin=[0.1]
  Math Function1 : Math  Operator=mod  SaturateOnIntegerOverflow=on
  PID Digital I 7 : MATLAB Function  TreatAsAtomicUnit=on
  Rate Transition7 : RateTransition  OutPortSampleTime=Ts_inv
  Sum : Sum  Inputs=|++
  Terminator1 : Terminator
  Terminator2 : Terminator
  Vq1 : Constant  Value=2*pi*fs  SampleTime=Ts_inv
  Vq2 : Constant  Value=0
  Vq6 : Constant  Value=2*pi  SampleTime=Ts_inv
  idq,inv2 : powerlib_meascontrol/Transformations/abc to dq0  Alignment=90 degrees behind phase A axis
  wt : Outport
  Freq : Outport  Port=2
  wires:
  Gain31/1 -> Analog Filter Design/1
  vabc,g/1 -> Rate Transition7/1
  idq,inv2/1 -> Dem_idq_LR2/1
  Vq6/1 -> Math Function1/2
  Discrete-Time Integrator/1 -> Math Function1/1
  Math Function1/1 -> wt/1, idq,inv2/2
  Vq2/1 -> PID Digital I 7/2(Med)
  Dem_idq_LR2/2 -> PID Digital I 7/1(Ref)
  Sum/1 -> Gain31/1, Discrete-Time Integrator/1
  Vq1/1 -> Sum/2
  PID Digital I 7/1(Out) -> Sum/1
  Constant1/1 -> PID Digital I 7/3(KI)
  Constant3/1 -> PID Digital I 7/4(KP)
  Dem_idq_LR2/3 -> Terminator1/1
  Dem_idq_LR2/1 -> Terminator2/1
  Rate Transition7/1 -> idq,inv2/1
  Analog Filter Design/1 -> Freq/1

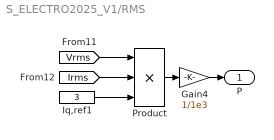
== system S_ELECTRO2025_V1/RMS ==
  Gain4 : Gain  Gain=1/1e3
  Iq,ref1 : Constant  Value=3  SampleTime=Ts4
  Product : Product  Inputs=3
  P : Outport
  wires:
  Gain4/1 -> P/1
  Product/1 -> Gain4/1
  Iq,ref1/1 -> Product/3
  [Vrms] -> Product/1
  [Irms] -> Product/2

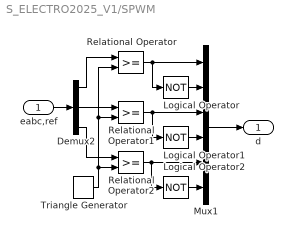
== system S_ELECTRO2025_V1/SPWM ==
  eabc,ref : Inport
  Demux2 : Demux  Outputs=3
  Logical Operator : Logic  Operator=NOT  AllPortsSameDT=off  OutDataTypeStr=boolean
  Logical Operator1 : Logic  Operator=NOT  AllPortsSameDT=off  OutDataTypeStr=boolean
  Logical Operator2 : Logic  Operator=NOT  AllPortsSameDT=off  OutDataTypeStr=boolean
  Mux1 : Mux  Inputs=6
  Relational Operator : RelationalOperator  OutDataTypeStr=boolean  RndMeth=Simplest
  Relational Operator1 : RelationalOperator  OutDataTypeStr=boolean  RndMeth=Simplest
  Relational Operator2 : RelationalOperator  OutDataTypeStr=boolean  RndMeth=Simplest
  Triangle Generator : powerlib_meascontrol/Pulse & Signal Generators/Triangle Generator  Freq=Fc  Phase=0  Ts=Ts_inv
  d : Outport
  wires:
  Logical Operator/1 -> Mux1/2
  Demux2/1 -> Relational Operator/1
  Demux2/2 -> Relational Operator1/1
  Logical Operator1/1 -> Mux1/4
  Relational Operator2/1 -> Mux1/5, Logical Operator2/1
  Triangle Generator/1 -> Relational Operator2/2, Relational Operator1/2, Relational Operator/2
  Mux1/1 -> d/1
  Relational Operator/1 -> Logical Operator/1, Mux1/1
  Logical Operator2/1 -> Mux1/6
  Demux2/3 -> Relational Operator2/1
  Relational Operator1/1 -> Logical Operator1/1, Mux1/3
  eabc,ref/1 -> Demux2/1

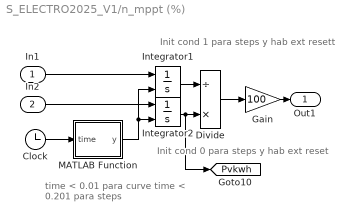
== system S_ELECTRO2025_V1/n_mppt (%) ==
  note: time < 0.01 para curve
      | time < 0.201 para steps
  note: Init cond 1 para steps y hab ext resett
  note: Init cond 0 para steps y hab ext reset
  In1 : Inport
  In2 : Inport  Port=2
  Clock : Clock
  Divide : Product  Inputs=/*
  Gain : Gain  Gain=100
  Integrator1 : Integrator  ExternalReset=level hold  InitialCondition=1  ZeroCross=off
  Integrator2 : Integrator  ExternalReset=level hold  ZeroCross=off
  MATLAB Function : MATLAB Function  TreatAsAtomicUnit=on
  Out1 : Outport
  tag scope: Pvkwh=global
  wires:
  In2/1 -> Integrator2/1
  Gain/1 -> Out1/1
  In1/1 -> Integrator1/1
  Integrator1/1 -> Divide/1
  Integrator2/1 -> [Pvkwh], Divide/2
  Divide/1 -> Gain/1
  Clock/1 -> MATLAB Function/1(time)
  MATLAB Function/1(y) -> Integrator1/2, Integrator2/2

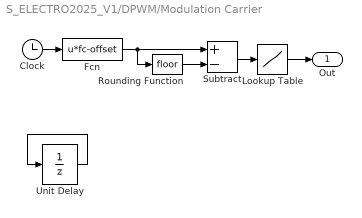
== system S_ELECTRO2025_V1/DPWM/Modulation Carrier ==
  Clock : Clock
  Fcn : Fcn  Expr=u*fc-offset
  Lookup Table : Lookup  InputValues=[0 .5 1]  Table=[range(1) range(2) range(1)]  LookUpMeth=Interpolation-Use End Values
  Rounding Function : Rounding
  Subtract : Sum  Inputs=+-
  Unit Delay : UnitDelay  SampleTime=si
  Out : Outport
  wires:
  Lookup Table/1 -> Out/1
  Subtract/1 -> Lookup Table/1
  Rounding Function/1 -> Subtract/2
  Fcn/1 -> Rounding Function/1, Subtract/1
  Clock/1 -> Fcn/1
  Unit Delay/1 -> Unit Delay/1

== matlab function S_ELECTRO2025_V1/Digital State Feedback Current Controller n_mppt = 88.18%, ta(2%) = 0.4 s con Steps de Irrad Interv. 2 Seg. n_mppt = 97.01%, ta(2%) = 0.1 s con Steps de Irrad Interv. 2 Seg. n_mppt = 86.2%, ta(2%) = 0.4 s con Steps de Irrad Interv. 0.5 Seg. n_mppt = 93.3%, ta(2%) = 0.1 s con Steps de Irrad Interv. 0.5 Seg. n_mppt = 96.15%, ta(2%) = 0.1 s con Curva de Irrad ta(2%) de 0.1 s se obtiene el ta de F-Tsukmam n_mppt = 89.31%, ta(2%) = 0.0692 s con Steps de Irrad Interv. 0.5 Seg. Menor ta y tr: mayor n_mppt pero genera mayor MP en id (impacto negativo PQ). Si se mantiene ta y se incrementa tr la n_mppt se mantiene al mismo tiempo que se mitigan los MP en id (impacto positivo en PQ)  /PID Digital I 1 ==
  data: x1_Ref input; x1 input; x2 input; UK output; Ki input; K1 input; K2 input; Ts input
function UK = fcn(x1_Ref, x1, x2, Ki, K1, K2, Ts)
    % Retroalimentación de estados con acción integral
    
    % Variables persistentes para mantener el estado entre llamadas
    persistent ek Acc_Int Acc_Int_1 uk
    
    if isempty(ek)
        ek = 0;
        Acc_Int = 0;
        Acc_Int_1 = 0;
        uk = 0;
    end

    % Cálculo del error
    ek = x1_Ref - x1;

    % Acción integral
    Acc_Int = Ki * ek * Ts + Acc_Int_1;
    Acc_Int_1 = Acc_Int;

    % Ley de control: acción integral menos retroalimentación de estados
    uk = Acc_Int - (K1 * x1 + K2 * x2);

    % Saturación (opcional)
    uk = min(max(uk, 0), 65535);

    % Salida del controlador
    UK = uk;
end

== matlab function S_ELECTRO2025_V1/Controladores del Inversor cd-ca/PID Digital I 1 ==
  data: IN_ref input; UK output; IN input; KI input; KP input
function UK = fcn(IN_ref, IN, KI, KP)

 %Valores iniciales de las conStantes del controlador
 persistent  ek uk
 persistent  ek_1 uk_1
 if isempty(ek)
    ek =0;
    uk =0;
    ek_1 =0;
    uk_1 =0;
 end
ek=IN_ref-IN;
uk=ek*(KP+KI)-ek_1*KP+uk_1;
if(uk>1000)
    uk=1000;
end
if(uk<-1000)
    uk=-1000;
end
ek_1=ek;
uk_1=uk;
UK=uk;
end

== matlab function S_ELECTRO2025_V1/Controladores del Inversor cd-ca/PID Digital I 2 ==
  data: IN_ref input; UK output; IN input; KI input; KP input
function UK = fcn(IN_ref, IN, KI, KP)

 %Valores iniciales de las conStantes del controlador
 persistent  ek uk
 persistent  ek_1 uk_1
 if isempty(ek)
    ek =0;
    uk =0;
    ek_1 =0;
    uk_1 =0;
 end
ek=IN_ref-IN;
uk=ek*(KP+KI)-ek_1*KP+uk_1;
if(uk>1000)
    uk=1000;
end
if(uk<-1000)
    uk=-1000;
end
ek_1=ek;
uk_1=uk;
UK=uk;
end

== matlab function S_ELECTRO2025_V1/Controladores del Inversor cd-ca/PID Digital I 3 ==
  data: IN_ref input; UK output; IN input; KI input; KP input
function UK = fcn(IN_ref, IN, KI, KP)

 %Valores iniciales de las conStantes del controlador
 persistent  ek uk
 persistent  ek_1 uk_1
 if isempty(ek)
    ek =0;
    uk =0;
    ek_1 =0;
    uk_1 =0;
 end
ek=IN_ref-IN;
uk=ek*(KP+KI)-ek_1*KP+uk_1;
if(uk>60)
    uk=60;
end
if(uk<-60)
    uk=-60;
end
ek_1=ek;
uk_1=uk;
UK=uk;
end

== matlab function S_ELECTRO2025_V1/PLL/PID Digital I 7 ==
  data: Ref input; Out output; Med input; KI input; KP input
function Out = fcn(Ref, Med, KI, KP)

 %Valores iniciales de las conStantes del controlador
 persistent  ek uk
 persistent  ek_1 uk_1
 if isempty(ek)
    ek =0;
    uk =0;
    ek_1 =0;
    uk_1 =0;
 end
ek=Ref-Med;
%uk=ek*(KP+KI)-ek_1*KP+uk_1;
uk=KP*ek+KI*ek+KI*ek_1;
ek_1=ek;
uk_1=uk;
Out=uk;
end

== matlab function S_ELECTRO2025_V1/n_mppt (%)/MATLAB Function ==
  data: y output; time input
function y = fcn(time)
    % Verifica si el valor es Inf
    if time < 0.201
        y = 1;  % Si es Inf, asigna 0
    else
        y = 0;  % Si no es Inf, devuelve el valor original
    end
end
